simulink model "forLoopTest"  (R2022a)
settings: Solver=VariableStepAuto  StartTime=0.0  StopTime=10.0  RelTol=1e-3
settings Model: Creator=targi  LastModifiedBy=targi

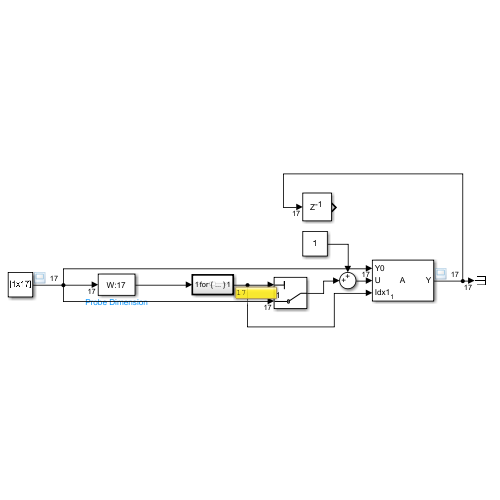
[thumbnail: Simulink's stored preview of the top-level diagram]
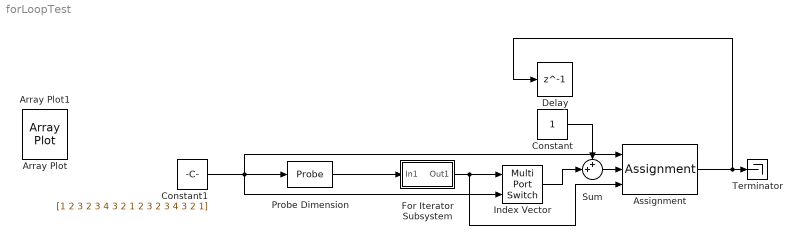
== system forLoopTest ==
  Assignment : Assignment  DiagnosticForDimensions=Warning  IndexOptions=Index vector (port)  Indices=1  OutputSizes=1
  Constant : Constant
  Constant1 : Constant  Value=[1 2 3 2 3 4 3 2 1 2 3 2 3 4 3 2 1]
  Delay : Delay  DelayLength=1  InitialCondition=0
  For Iterator Subsystem : Subsystem  TreatAsAtomicUnit=on
  Index Vector : MultiPortSwitch  Inputs=1  SaturateOnIntegerOverflow=off  InputSameDT=off
  Probe Dimension : Probe  ProbeSampleTime=off  ProbeComplexSignal=off
  Sum : Sum  Inputs=++|
  Terminator : Terminator
  Array Plot : ArrayPlot  IOType=viewer  WindowPosition=[699.000000,462.000000,800.000000,500.000000,]  IsFloating=on  ScopeFrameLocation=window  YLimits=[0.625,4.375]  DefaultConfigurationName=dsp.scopes.ArrayPlotBlockSpecification
  Array Plot1 : ArrayPlot  IOType=viewer  WindowPosition=[38.000000,463.000000,800.000000,500.000000,]  IsFloating=on  ScopeFrameLocation=window  YLimits=[0.625,4.375]  DefaultConfigurationName=dsp.scopes.ArrayPlotBlockSpecification
  wires:
  Probe Dimension/1 -> For Iterator Subsystem/1(In1)
  For Iterator Subsystem/1(Out1) -> Assignment/3, Index Vector/1
  Constant1/1 -> Index Vector/2, Assignment/1, Probe Dimension/1
  Sum/1 -> Assignment/2
  Index Vector/1 -> Sum/2
  Constant/1 -> Sum/1
  Assignment/1 -> Delay/1, Terminator/1

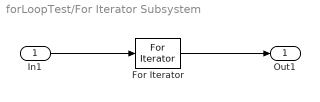
== system forLoopTest/For Iterator Subsystem ==
  In1 : Inport
  For Iterator : ForIterator  IterationSource=external
  Out1 : Outport
  wires:
  In1/1 -> For Iterator/1
  For Iterator/1 -> Out1/1
